simulink model "controller_node"  (R2020a)
settings: Solver=FixedStepAuto  StartTime=0.0  StopTime=inf  RelTol=1e-3
PreLoadFcn:
  | % ROS setup
  | rosshutdown;
  | ipAddr = '';
  | rosinit(ipAddr)
  | 
  | % Sample times
  | sampleTime = 0.2;
  | 
  | % Control parameters
  | ctrlParam1 = 2;
  | ctrlParam2 = 3.5;
undefined symbols (not defined in the file or in its folder): Rudder, Winch
libraries: robotlib x5, UBCSailbotBlocks x1
settings Model: Creator=scastro  LastModifiedBy=bruce
settings DataIOCC: ReturnWorkspaceOutputs=off
settings OptimizationCC: PassReuseOutputArgsAs=Individual arguments  MaxStackSize=64  EfficientTunableParamExpr=on
settings DebuggingCC: ParameterTunabilityLossMsg=error  ArithmeticOperatorsInVariantConditions=warning
settings HardwareCC: ProdBitPerPointer=32  ProdBitPerSizeT=32  ProdBitPerPtrDiffT=32  ProdLargestAtomicFloat=None  ProdIntDivRoundTo=Undefined  ProdEndianess=Unspecified  ProdWordSize=32  ProdHWDeviceType=Generic->Unspecified (assume 32-bit Generic)
settings SFSimCC: SimUseLocalCustomCode=off  MATLABDynamicMemAlloc=off  CustomCodeUndefinedFunction=UseInterfaceOnly
settings RTWCC: SystemTargetFile=ert.tlc  HardwareBoard=Robot Operating System (ROS)  TemplateMakefile=ert_default_tmf  GenerateReport=on  RTWUseLocalCustomCode=off  Toolchain=Catkin  IncludeHyperlinkInReport=on  LaunchReport=on  TargetLang=C++  GenerateTraceInfo=on  GenerateTraceReport=on  GenerateTraceReportSl=on  GenerateTraceReportSf=on  GenerateTraceReportEml=on
settings CodeAppCC: ForceParamTrailComments=on  IgnoreCustomStorageClasses=off  OperatorAnnotations=on  SimulinkDataObjDesc=on  SFDataObjDesc=on  InsertBlockDesc=on
settings ERTTargetCC: SupportContinuousTime=on

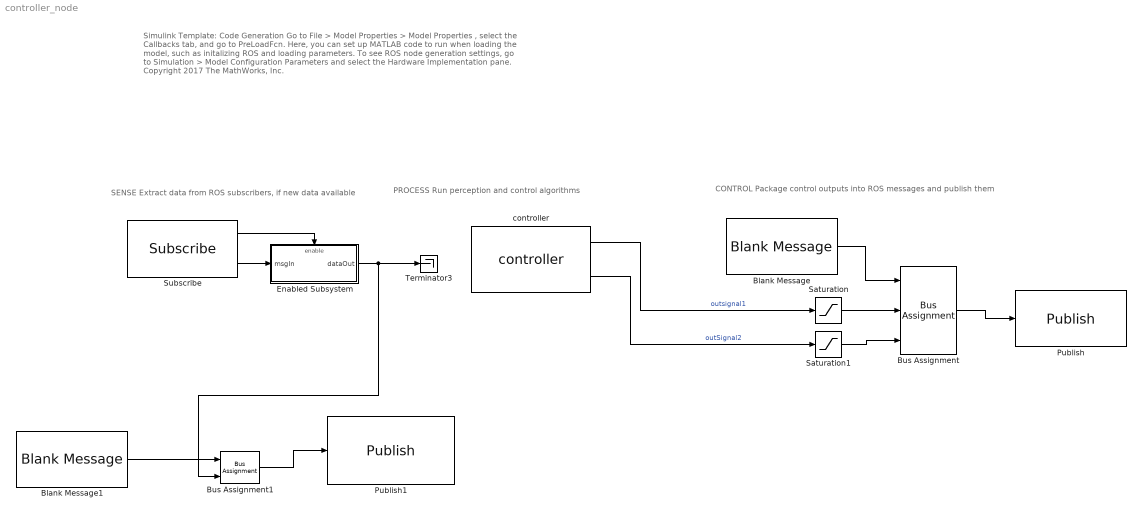
== system controller_node ==
  note: PROCESS
      | Run perception and control algorithms
  note: SENSE
      | Extract data from ROS subscribers, if new data available
  note: CONTROL
      | Package control outputs into ROS messages and publish them
  note: Simulink Template: Code Generation
      |
      | Go to File > Model Properties > Model Properties , select the Callbacks tab, and go to PreLoadFcn. Here, you can set up MATLAB code to run when loading the model, such as initalizing ROS and loading parameters.
      |
      | To see ROS node generation settings, go to Simulation > Model Configuration Parameters and select the Hardware Implementation pane.
      |
      | Copyright 2017 The MathWorks, Inc.
  Blank Message : robotlib/Blank Message  messageClass=Message  entityType=sailbot_msg/actuation_angle  messageType=sailbot_msg/actuation_angle  SampleTime=inf
  Blank Message1 : robotlib/Blank Message  messageClass=Message  entityType=std_msgs/Int32  messageType=std_msgs/Int32  SampleTime=inf
  Bus Assignment : BusAssignment  AssignedSignals=Rudder,Winch
  Bus Assignment1 : BusAssignment  AssignedSignals=Data
  Enabled Subsystem : Subsystem  TreatAsAtomicUnit=on
  Publish : robotlib/Publish  topicSource=Specify your own  topic=/actuation_angles  messageType=sailbot_msg/actuation_angle  messageQueueLength=1
  Publish1 : robotlib/Publish  topicSource=Specify your own  topic=/test_correct_subscribe_sensors  messageType=std_msgs/Int32  messageQueueLength=1
  Saturation : Saturate  UpperLimit=pi/3  LowerLimit=-pi/3
  Saturation1 : Saturate  UpperLimit=pi/2  LowerLimit=0
  Subscribe : robotlib/Subscribe  topicSource=Specify your own  topic=/sensors  messageType=sailbot_msg/Sensors  sampleTime=-1  messageQueueLength=1
  Terminator3 : Terminator
  controller : UBCSailbotBlocks/controller  SystemSampleTime=-1  Latency=0  AutoFrameSizeCalculation=off
  wires:
  Subscribe/2 -> Enabled Subsystem/1(msgIn)
  Subscribe/1 -> Enabled Subsystem/Enable
  Bus Assignment/1 -> Publish/1
  Blank Message/1 -> Bus Assignment/1
  controller/1 -> Saturation/1  "outsignal1"
  controller/2 -> Saturation1/1  "outSignal2"
  Saturation/1 -> Bus Assignment/2
  Saturation1/1 -> Bus Assignment/3
  Blank Message1/1 -> Bus Assignment1/1
  Enabled Subsystem/1(dataOut) -> Terminator3/1, Bus Assignment1/2
  Bus Assignment1/1 -> Publish1/1

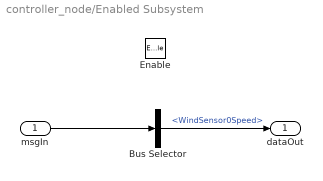
== system controller_node/Enabled Subsystem ==
  msgIn : Inport
  Enable : EnablePort
  Bus Selector : BusSelector  OutputSignals=WindSensor0Speed
  dataOut : Outport  VectorParamsAs1DForOutWhenUnconnected=off
  wires:
  msgIn/1 -> Bus Selector/1
  Bus Selector/1 -> dataOut/1  "<WindSensor0Speed>"
